simulink model "GCI_Ctrl_PLL_C2000"  (R2024a)
settings: Solver=FixedStepDiscrete  StartTime=0.0  StopTime=8  FixedStep=Sim.ContSampleTime  RelTol=1e-3  EnableMultiTasking=on
values from neighbouring files (symbols this model uses):
  ADPTV = 1.3912    [ModelDD.sldd]
  Ctrl = 0    [ModelDD.sldd]
  EnableMonitors = 0    [ModelDD.sldd]
  FrcPwr = 1    [ModelDD.sldd]
  IdSp = 0.0    [ModelDD.sldd]
  IqSp = 0.0    [ModelDD.sldd]
  ModReq = 1    [ModelDD.sldd]
  PorISel = 0    [ModelDD.sldd]
  PSp = 0.0    [ModelDD.sldd]
  QSp = 0.0    [ModelDD.sldd]
  Sim : value not decoded    [ModelDD.sldd]
  Test = 0    [ModelDD.sldd]
  Var = 650.0    [ModelDD.sldd]
undefined symbols (not defined in the file or in its folder): DiscIntNeverNeededParam, Down, GPTRIP1SEL, GPTRIP2SEL, magnitude, P, TZ1, TZ2, Up
libraries: simulink x38, c2837xDlib x22, c2802xlib x15, slpidlib x9, spsMeanLib x9, spsCurrentMeasurementLib x7, spsThreePhaseVIMeasurementLib x5, spsVoltageMeasurementLib x5, spsTHDLib x4, spsSeriesRLCBranchLib x4, svdutilitieslib x3, c280xlib x3
(part 1 of 11)
settings Model: SimulationMode=accelerator  ExtModeTrigDuration=8  Creator=OmarH  LastModifiedBy=The Professionals
settings SolverCC: AlgebraicLoopSolver=TrustRegion
settings DataIOCC: SaveFormat=StructureWithTime  SaveOutput=off  DSMLogging=off  SaveTime=off
settings OptimizationCC: DefaultParameterBehavior=Inlined  DefaultUnderspecifiedDataType=single  EnhancedBackFolding=on  PassReuseOutputArgsAs=Individual arguments  EfficientMapNaN2IntZero=off  MaxStackSize=1024  OptimizeBlockOrder=speed  DifferentSizesBufferReuse=on  OptimizationCustomize=off  DenormalBehavior=FlushToZero  EfficientTunableParamExpr=on
settings DebuggingCC: MultiTaskDSMMsg=none  ParameterTunabilityLossMsg=error  UnconnectedInputMsg=warning  UnconnectedOutputMsg=warning  UnconnectedLineMsg=warning
settings HardwareCC: ProdBitPerChar=16  ProdBitPerInt=16  ProdBitPerPointer=32  ProdBitPerSizeT=32  ProdBitPerPtrDiffT=32  ProdLargestAtomicInteger=Integer  ProdLargestAtomicFloat=None  ProdWordSize=16  ProdLongLongMode=on  ProdHWDeviceType=Texas Instruments->C2000  TargetBitPerChar=16  TargetBitPerInt=16  TargetLargestAtomicInteger=Integer  TargetIntDivRoundTo=Zero  TargetEndianess=LittleEndian  TargetWordSize=16  TargetHWDeviceType=Texas Instruments->C2000  HardwareBoardFeatureSet=SoCBlockset
settings ModelReferenceCC: EnableRefExpFcnMdlSchedulingChecks=on  ModelReferenceNumInstancesAllowed=Single
settings SFSimCC: MATLABDynamicMemAlloc=off
settings RTWCC: Description=Embedded Coder  SystemTargetFile=ert.tlc  HardwareBoard=TI Delfino F28379D LaunchPad  TemplateMakefile=ert_default_tmf  Toolchain=Texas Instruments Code Composer Studio (C2000)  CodeProfilingSaveOptions=MetricsOnly
settings CodeAppCC: ForceParamTrailComments=on  IgnoreCustomStorageClasses=off  MaxIdLength=128  OperatorAnnotations=on  SimulinkDataObjDesc=on  SFDataObjDesc=on  InsertBlockDesc=on
settings ERTTargetCC: CodeReplacementLibrary=TI C28x  ExtMode=on  ExtModeTransport=4  ExtModeStaticAlloc=on  ExtModeAutomaticAllocSize=off  ExtModeStaticAllocSize=10000  ExtModeMexFile=ext_xcp  ExtModeMexArgs=1 4 5000000  ExtModeIntrfLevel=Level2 - Open

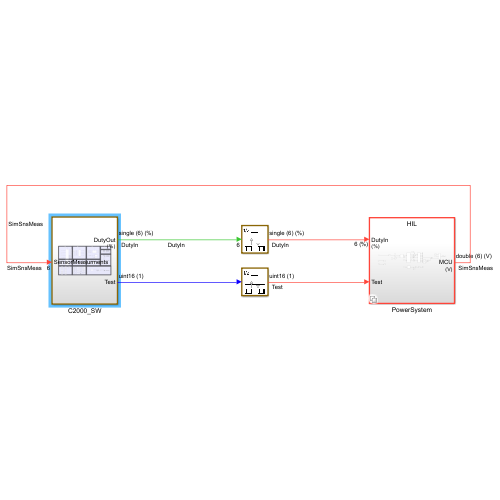
[thumbnail: Simulink's stored preview of the top-level diagram]
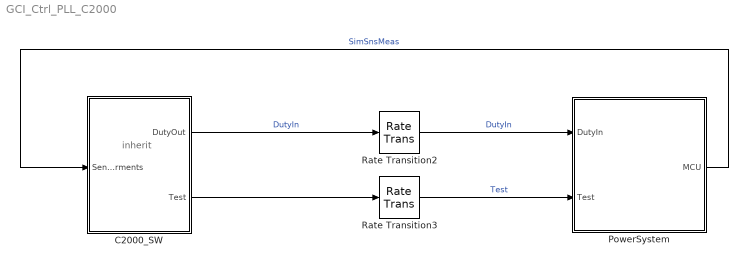
== system GCI_Ctrl_PLL_C2000 ==
  note: inherit
  C2000_SW : Subsystem
  PowerSystem : Subsystem  Variant=on  VariantControl=Variant1
  Rate Transition2 : RateTransition  OutPortSampleTime=Sim.ContSampleTime
  Rate Transition3 : RateTransition  OutPortSampleTime=Sim.ContSampleTime
  wires:
  Rate Transition3/1 -> PowerSystem/2(Test)  "Test"
  C2000_SW/2(Test) -> Rate Transition3/1
  PowerSystem/1(MCU) -> C2000_SW/1(SensorMeasurments)  "SimSnsMeas"
  C2000_SW/1(DutyOut) -> Rate Transition2/1  "DutyIn"
  Rate Transition2/1 -> PowerSystem/1(DutyIn)  "DutyIn"

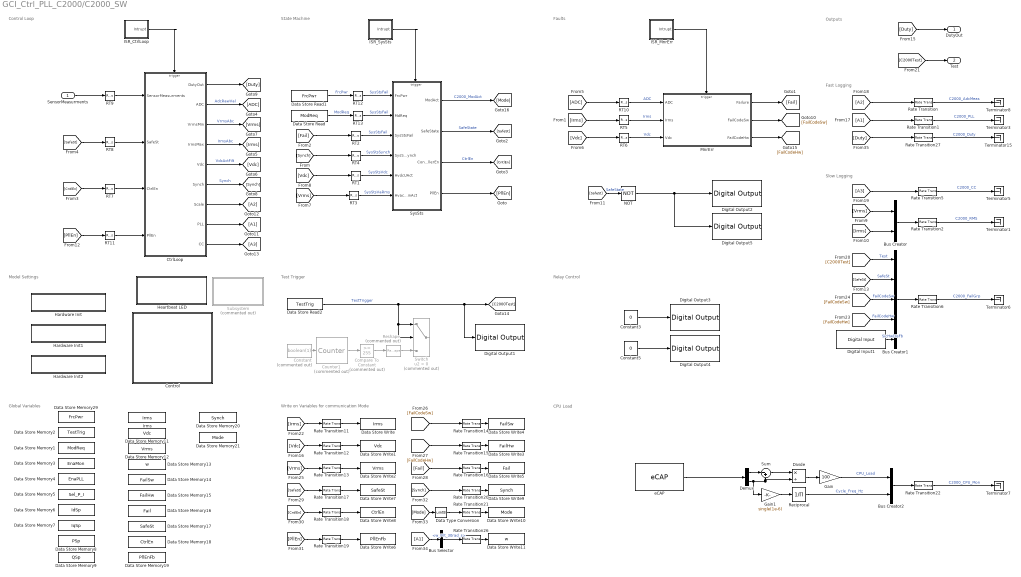
== system GCI_Ctrl_PLL_C2000/C2000_SW ==
  note: Model Settings
  note: Write on Variables for communication Mode
  note: Global Variables
  note: CPU Load
  note: Outputs
  note: Test Trigger
  note: Faults
  note: Relay Control
  note: Control Loop
  note: State Machine
  note: Fast Logging
  note: Slow Logging
  SensorMeasurments : Inport
  Bus Creator : BusCreator  Inputs=2
  Bus Creator1 : BusCreator  Inputs=5
  Bus Creator2 : BusCreator  Inputs=2
  Bus Selector : BusSelector  OutputSignals=w_Filt_30rad_s
  Compare To Constant : simulink/Logic and Bit Operations/Compare To Constant  Commented=on  relop=>=  const=255  OutDataTypeStr=boolean
  Constant : Constant  Commented=on  Value=boolean(1)
  Constant3 : Constant  Value=0  OutDataTypeStr=boolean  SampleTime=10/double(Var.PWM_Freq)
  Constant5 : Constant  Value=0  OutDataTypeStr=boolean  SampleTime=10/double(Var.PWM_Freq)
  Control : Subsystem  Variant=on  VariantControl=Subsystem1
  Counter1 : dspswit3/Counter  Commented=on  Direction=Up  CountEvent=Free running  CounterSize=8 bits  MaxCount=255  InitialCount=0  Output=Count  HitValue=32  ResetInput=on  SamplesPerFrame=1  Ts=1  CntDtype=uint8  HitDtype=Logical
  CtrlLoop : Subsystem
  Data Store Memory1 : DataStoreMemory  DataStoreName=ModReq  WriteAfterWriteMsg=warning  ShowAdditionalParam=off
  Data Store Memory11 : DataStoreMemory  DataStoreName=Vdc  WriteAfterWriteMsg=warning  WriteAfterReadMsg=warning  ShowAdditionalParam=off  OutDataTypeStr=single
  Data Store Memory12 : DataStoreMemory  DataStoreName=Vrms  WriteAfterWriteMsg=warning  WriteAfterReadMsg=warning  ShowAdditionalParam=off  OutDataTypeStr=single
  Data Store Memory13 : DataStoreMemory  DataStoreName=w  WriteAfterWriteMsg=warning  WriteAfterReadMsg=warning  ShowAdditionalParam=off  OutDataTypeStr=single
  Data Store Memory14 : DataStoreMemory  DataStoreName=FailSw  WriteAfterWriteMsg=warning  WriteAfterReadMsg=warning  ShowAdditionalParam=off  OutDataTypeStr=uint16
  Data Store Memory15 : DataStoreMemory  DataStoreName=FailHw  WriteAfterWriteMsg=warning  WriteAfterReadMsg=warning  ShowAdditionalParam=off  OutDataTypeStr=uint8
  Data Store Memory16 : DataStoreMemory  DataStoreName=Fail  WriteAfterWriteMsg=warning  WriteAfterReadMsg=warning  ShowAdditionalParam=off  OutDataTypeStr=boolean
  Data Store Memory17 : DataStoreMemory  DataStoreName=SafeSt  WriteAfterWriteMsg=warning  WriteAfterReadMsg=warning  ShowAdditionalParam=off  OutDataTypeStr=boolean
  Data Store Memory18 : DataStoreMemory  DataStoreName=CtrlEn  WriteAfterWriteMsg=warning  WriteAfterReadMsg=warning  ShowAdditionalParam=off  OutDataTypeStr=boolean
  Data Store Memory19 : DataStoreMemory  DataStoreName=PllEnFb  WriteAfterWriteMsg=warning  WriteAfterReadMsg=warning  ShowAdditionalParam=off  OutDataTypeStr=boolean
  Data Store Memory2 : DataStoreMemory  DataStoreName=TestTrig  WriteAfterWriteMsg=warning  WriteAfterReadMsg=warning  ShowAdditionalParam=off
  Data Store Memory20 : DataStoreMemory  DataStoreName=Synch  WriteAfterWriteMsg=warning  WriteAfterReadMsg=warning  ShowAdditionalParam=off  OutDataTypeStr=boolean
  Data Store Memory21 : DataStoreMemory  DataStoreName=Mode  WriteAfterWriteMsg=warning  WriteAfterReadMsg=warning  ShowAdditionalParam=off  OutDataTypeStr=uint8
  Data Store Memory29 : DataStoreMemory  DataStoreName=FrcPwr  WriteAfterWriteMsg=warning  ShowAdditionalParam=off
  Data Store Memory3 : DataStoreMemory  DataStoreName=EnaMon  ShowAdditionalParam=off
  Data Store Memory4 : DataStoreMemory  DataStoreName=EnaPLL  WriteAfterWriteMsg=warning  WriteAfterReadMsg=warning  ShowAdditionalParam=off  OutDataTypeStr=boolean
  Data Store Memory5 : DataStoreMemory  DataStoreName=Sel_P_I  ShowAdditionalParam=off
  Data Store Memory6 : DataStoreMemory  DataStoreName=IdSp  ShowAdditionalParam=off  OutDataTypeStr=single
  Data Store Memory7 : DataStoreMemory  DataStoreName=IqSp  ShowAdditionalParam=off  OutDataTypeStr=single
  Data Store Memory8 : DataStoreMemory  DataStoreName=PSp  WriteAfterWriteMsg=warning  ShowAdditionalParam=off  OutDataTypeStr=single
  Data Store Memory9 : DataStoreMemory  DataStoreName=QSp  WriteAfterWriteMsg=warning  ShowAdditionalParam=off  OutDataTypeStr=single
  Data Store Read : DataStoreRead  DataStoreName=ModReq  SampleTime=10/double(Var.PWM_Freq)  IndexOptions=Index vector (dialog)  Indices=1  OutputSizes=1
  Data Store Read1 : DataStoreRead  DataStoreName=FrcPwr  SampleTime=10/double(Var.PWM_Freq)  IndexOptions=Index vector (dialog)  Indices=1  OutputSizes=1
  Data Store Read2 : DataStoreRead  DataStoreName=TestTrig  SampleTime=10/double(Var.PWM_Freq)  IndexOptions=Index vector (dialog)  Indices=1  OutputSizes=1
  Data Store Write : DataStoreWrite  DataStoreName=Irms  IndexOptions=Index vector (dialog)  Indices=1  OutputSizes=1
  Data Store Write1 : DataStoreWrite  DataStoreName=Vdc  IndexOptions=Index vector (dialog)  Indices=1  OutputSizes=1
  Data Store Write10 : DataStoreWrite  DataStoreName=Mode  IndexOptions=Index vector (dialog)  Indices=1  OutputSizes=1
  Data Store Write11 : DataStoreWrite  DataStoreName=w  IndexOptions=Index vector (dialog)  Indices=1  OutputSizes=1
  Data Store Write2 : DataStoreWrite  DataStoreName=Vrms  IndexOptions=Index vector (dialog)  Indices=1  OutputSizes=1
  Data Store Write3 : DataStoreWrite  DataStoreName=FailHw  IndexOptions=Index vector (dialog)  Indices=1  OutputSizes=1
  Data Store Write4 : DataStoreWrite  DataStoreName=FailSw  IndexOptions=Index vector (dialog)  Indices=1  OutputSizes=1
  Data Store Write5 : DataStoreWrite  DataStoreName=Fail  IndexOptions=Index vector (dialog)  Indices=1  OutputSizes=1
  Data Store Write6 : DataStoreWrite  DataStoreName=PllEnFb  IndexOptions=Index vector (dialog)  Indices=1  OutputSizes=1
  Data Store Write7 : DataStoreWrite  DataStoreName=SafeSt  IndexOptions=Index vector (dialog)  Indices=1  OutputSizes=1
  Data Store Write8 : DataStoreWrite  DataStoreName=CtrlEn  IndexOptions=Index vector (dialog)  Indices=1  OutputSizes=1
  Data Store Write9 : DataStoreWrite  DataStoreName=Synch  IndexOptions=Index vector (dialog)  Indices=1  OutputSizes=1
  Data Type Conversion : DataTypeConversion  OutDataTypeStr=uint8  SaturateOnIntegerOverflow=off  RndMeth=Floor
  Demux : Demux  Outputs=2
  Digital Input1 : c2837xDlib/Digital Input  GPIO_Number=GPIO88~GPIO95  GPIO_Bit0=off  GPIO_Bit1=off  GPIO_Bit2=off  GPIO_Bit3=off  GPIO_Bit4=off  GPIO_Bit5=off  GPIO_Bit6=on  GPIO_Bit7=off  sampleTime=10/double(Var.PWM_Freq)  dataType=boolean  GPIO_Bit0_Qualification=Sync to SYSCLKOUT  GPIO_Bit1_Qualification=Sync to SYSCLKOUT  GPIO_Bit2_Qualification=Sync to SYSCLKOUT  GPIO_Bit3_Qualification=Sync to SYSCLKOUT  GPIO_Bit4_Qualification=Sync to SYSCLKOUT  GPIO_Bit5_Qualification=Sync to SYSCLKOUT  GPIO_Bit6_Qualification=Sync to SYSCLKOUT  GPIO_Bit7_Qualification=Sync to SYSCLKOUT  Qualification_Period=-1
  Digital Output1 : c2837xDlib/Digital Output  GPIO_Number=GPIO64~GPIO71  GPIO_Bit0=off  GPIO_BIT0_Toggle=off  GPIO_Bit1=off  GPIO_BIT1_Toggle=off  GPIO_Bit2=off  GPIO_BIT2_Toggle=off  GPIO_Bit3=on  GPIO_BIT3_Toggle=off  GPIO_Bit4=off  GPIO_BIT4_Toggle=off  GPIO_Bit5=off  GPIO_BIT5_Toggle=off  GPIO_Bit6=off  GPIO_BIT6_Toggle=off  GPIO_Bit7=off  GPIO_BIT7_Toggle=off
  Digital Output2 : c2837xDlib/Digital Output  GPIO_Number=GPIO8~GPIO15  GPIO_Bit0=off  GPIO_BIT0_Toggle=off  GPIO_Bit1=off  GPIO_BIT1_Toggle=off  GPIO_Bit2=off  GPIO_BIT2_Toggle=off  GPIO_Bit3=off  GPIO_BIT3_Toggle=off  GPIO_Bit4=on  GPIO_BIT4_Toggle=off  GPIO_Bit5=off  GPIO_BIT5_Toggle=off  GPIO_Bit6=off  GPIO_BIT6_Toggle=off  GPIO_Bit7=off  GPIO_BIT7_Toggle=off
  Digital Output3 : c2837xDlib/Digital Output  GPIO_Number=GPIO16~GPIO23  GPIO_Bit0=off  GPIO_BIT0_Toggle=off  GPIO_Bit1=off  GPIO_BIT1_Toggle=off  GPIO_Bit2=on  GPIO_BIT2_Toggle=off  GPIO_Bit3=off  GPIO_BIT3_Toggle=off  GPIO_Bit4=off  GPIO_BIT4_Toggle=off  GPIO_Bit5=off  GPIO_BIT5_Toggle=off  GPIO_Bit6=off  GPIO_BIT6_Toggle=off  GPIO_Bit7=off  GPIO_BIT7_Toggle=off
  Digital Output4 : c2837xDlib/Digital Output  GPIO_Number=GPIO16~GPIO23  GPIO_Bit0=off  GPIO_BIT0_Toggle=off  GPIO_Bit1=off  GPIO_BIT1_Toggle=off  GPIO_Bit2=off  GPIO_BIT2_Toggle=off  GPIO_Bit3=on  GPIO_BIT3_Toggle=off  GPIO_Bit4=off  GPIO_BIT4_Toggle=off  GPIO_Bit5=off  GPIO_BIT5_Toggle=off  GPIO_Bit6=off  GPIO_BIT6_Toggle=off  GPIO_Bit7=off  GPIO_BIT7_Toggle=off
  Digital Output5 : c2837xDlib/Digital Output  GPIO_Number=GPIO8~GPIO15  GPIO_Bit0=off  GPIO_BIT0_Toggle=off  GPIO_Bit1=off  GPIO_BIT1_Toggle=off  GPIO_Bit2=off  GPIO_BIT2_Toggle=off  GPIO_Bit3=off  GPIO_BIT3_Toggle=off  GPIO_Bit4=off  GPIO_BIT4_Toggle=off  GPIO_Bit5=off  GPIO_BIT5_Toggle=off  GPIO_Bit6=on  GPIO_BIT6_Toggle=off  GPIO_Bit7=off  GPIO_BIT7_Toggle=off
  Divide : Product  Inputs=*/
  Gain : Gain  Gain=100
  Gain1 : Gain  Gain=single(1e-6)  ParamDataTypeStr=single
  Hardware Init : Subsystem  TreatAsAtomicUnit=on
  Hardware Init1 : Subsystem  TreatAsAtomicUnit=on
  Hardware Init2 : Subsystem  TreatAsAtomicUnit=on
  Heartbeat LED : Subsystem
  ISR_CtrlLoop : Subsystem  Variant=on  VariantControl=Variant1
  ISR_MnrErr : Subsystem  Variant=on  VariantControl=Variant1
  ISR_SysSts : Subsystem  Variant=on  VariantControl=Variant1
  Irms : DataStoreMemory  DataStoreName=Irms  WriteAfterWriteMsg=warning  WriteAfterReadMsg=warning  ShowAdditionalParam=off  OutDataTypeStr=single
  MnrErr : Subsystem
  NOT : Logic  Operator=NOT  IconShape=distinctive  AllPortsSameDT=off  OutDataTypeStr=boolean
  RT{1..13} (13 alike) : RateTransition  Deterministic=off  OutPortSampleTimeOpt=Inherit  OutPortSampleTime=0.001
  Rate Transition : RateTransition  Deterministic=off  OutPortSampleTime=Sim.MeasFastSmplTime
  Rate Transition1 : RateTransition  Deterministic=off  OutPortSampleTime=Sim.MeasFastSmplTime
  Rate Transition{2,5..6,11..22,26} (16 alike) : RateTransition  Deterministic=off  OutPortSampleTime=Sim.MeasSlowSmplTime
  Rate Transition27 : RateTransition  Deterministic=off  OutPortSampleTime=Sim.MeasFastSmplTime
  Reciprocal : Product  Inputs=/
  Reshape : Reshape  Commented=on
  Subsystem : Subsystem  Commented=on
  Sum : Sum  Inputs=|-+
  Switch : Switch  Commented=on  Criteria=u2 > Threshold  SaturateOnIntegerOverflow=off  InputSameDT=off
  SysSts : Subsystem
  Terminator{1,3,5..8,15} (7 alike) : Terminator
  eCAP : c280xlib/eCAP  operatingMode=eCAP  selectCAPx=eCAP1  offsetValue=0  counterSynIn=off  enableCounter=off  syncOutput=Disabled  sampleTime=1/1000  eventPrescaler=0  HREnable=off  continuousCalibration=off  calibrationPeriod=0.0016  selectMode=Continuous  enableOneShot=off  stopValue=Capture Event 2  resetEv1Ts=off  ev1Polarity=Rising Edge  resetEv2Ts=on  ev2Polarity=Falling Edge  resetEv3Ts=off  ev3Polarity=Rising Edge  resetEv4Ts=off  ev4Polarity=Rising Edge  outputType=Microseconds  tSCntrDataType=single  capEvFlag=off  capFlagDataType=uint16  overFlowFlag=off  overFlowFlagDataType=uint16  periodUnit=Seconds  periodSource=Specify via dialog  waveformPeriod=0.001  dutyUnit=Percentages  dutySource=Specify via dialog  dutyCycle=50  outputPolarity=Active High  enableCEVT1Int=off  enableCEVT2Int=off  enableCEVT3Int=off  enableCEVT4Int=off  enableCTROVFInt=off  enablePRDInt=off  enableCMPInt=off
      settings: LibrarySourceBlock=c2837xDlib/eCAP
  DutyOut : Outport  Unit=%
  Test : Outport  Port=2
  wires:
  ISR_CtrlLoop/1(Intrupt) -> CtrlLoop/Trigger
  ISR_SysSts/1(Intrupt) -> SysSts/Trigger
  MnrErr/1(Failure) -> [Fail]
  Data Store Read/1 -> RT13/1  "ModReq"
  [SafeSt] -> RT8/1
  [CntlEn] -> RT7/1
  ISR_MnrErr/1(Intrupt) -> MnrErr/Trigger
  CtrlLoop/2(ADC) -> [ADC]  "AdcRawVal"
  CtrlLoop/4(IrmsMax) -> [Irms]  "IrmsAbc"
  [Irms] -> RT5/1
  [Vdc] -> RT6/1
  CtrlLoop/3(VrmsMin) -> [Vrms]  "VrmsAbc"
  RT3/1 -> SysSts/6(HvacUMinAct)  "SysStsVaRms"
  [Vrms] -> RT3/1
  [Vdc] -> RT1/1
  [Fail] -> RT2/1
  RT10/1 -> MnrErr/1(ADC)  "ADC"
  RT5/1 -> MnrErr/2(Irms)  "Irms"
  RT6/1 -> MnrErr/3(Vdc)  "Vdc"
  CtrlLoop/6(Synch) -> [Synch]  "Synch"
  [Synch] -> RT4/1
  Data Store Read1/1 -> RT12/1  "FrcPwr"
  [ADC] -> RT10/1
  RT4/1 -> SysSts/4(SysStsSynch)  "SysStsSynch"
  RT1/1 -> SysSts/5(HvdcUAct)  "SysStsVdc"
  RT2/1 -> SysSts/3(SysStsFail)  "SysStsFail"
  SysSts/2(SafeState) -> [SafeSt]  "SafeState"
  SysSts/3(ControllerEn) -> [CntlEn]  "CtrlEn"
  CtrlLoop/5(Vdc) -> [Vdc]  "VdcActFilt"
  Rate Transition/1 -> Terminator8/1  "C2000_AdcMeas"
  Rate Transition1/1 -> Terminator3/1  "C2000_PLL"
  Rate Transition2/1 -> Terminator1/1  "C2000_RMS"
  CtrlLoop/1(DutyOut) -> [Duty]
  Rate Transition5/1 -> Terminator5/1  "C2000_CC"
  Counter1/1 -> Compare To Constant/1
  Compare To Constant/1 -> Reshape/1
  Rate Transition6/1 -> Terminator6/1  "C2000_FailGrp"
  RT7/1 -> CtrlLoop/3(CtrlEn)
  RT8/1 -> CtrlLoop/2(SafeSt)
  [SafeSt] -> NOT/1  "SafeState"
  SensorMeasurments/1 -> RT9/1
  RT9/1 -> CtrlLoop/1(SensorMeasurments)
  SysSts/1(ModAct) -> [Mode]  "C2000_ModAct"
  RT11/1 -> CtrlLoop/4(PllEn)
  [PllEn] -> RT11/1
  SysSts/4(PllEn) -> [PllEn]
  Reshape/1 -> Switch/3
  [Duty] -> DutyOut/1
  CtrlLoop/8(PLL) -> [A1]
  [A1] -> Rate Transition1/1
  CtrlLoop/7(" Scale") -> [A2]
  [A2] -> Rate Transition/1
  CtrlLoop/9(CC) -> [A3]
  [A3] -> Rate Transition5/1
  [C2000Test] -> Test/1
  MnrErr/2(FailCodeSw) -> [FailCodeSw]
  Constant5/1 -> Digital Output4/1
  Constant3/1 -> Digital Output3/1
  MnrErr/3(FailCodeHw) -> [FailCodeHw]
  NOT/1 -> Digital Output5/1, Digital Output2/1
  Constant/1 -> Counter1/1
  Rate Transition22/1 -> Terminator7/1  "C2000_CPU_Mon"
  eCAP/1 -> Demux/1
  Demux/1 -> Sum/1
  Demux/2 -> Gain1/1, Sum/2, Divide/2
  Sum/1 -> Divide/1
  Divide/1 -> Gain/1
  Gain/1 -> Bus Creator2/1  "CPU_Load"
  Reciprocal/1 -> Bus Creator2/2  "Cycle_Freq_Hz"
  Gain1/1 -> Reciprocal/1
  Data Store Read2/1 -> Switch/1, Switch/2, Digital Output1/1, [C2000Test]  "TestTrigger"
  Rate Transition21/1 -> Data Store Write10/1
  [CntlEn] -> Rate Transition18/1
  [FailCodeHw] -> Rate Transition15/1
  [Synch] -> Rate Transition20/1
  [PllEn] -> Rate Transition19/1
  Rate Transition18/1 -> Data Store Write8/1
  Rate Transition19/1 -> Data Store Write6/1
  [FailCodeSw] -> Rate Transition14/1
  Rate Transition16/1 -> Data Store Write5/1
  [SafeSt] -> Rate Transition17/1
  Rate Transition14/1 -> Data Store Write4/1
  [Mode] -> Data Type Conversion/1
  Rate Transition20/1 -> Data Store Write9/1
  Rate Transition17/1 -> Data Store Write7/1
  Rate Transition15/1 -> Data Store Write3/1
  Rate Transition12/1 -> Data Store Write1/1
  Rate Transition11/1 -> Data Store Write/1
  [Vrms] -> Rate Transition13/1
  Data Type Conversion/1 -> Rate Transition21/1
  Rate Transition13/1 -> Data Store Write2/1
  [Fail] -> Rate Transition16/1
  [Vdc] -> Rate Transition12/1
  [Irms] -> Rate Transition11/1
  Bus Selector/1 -> Rate Transition26/1  "<w_Filt_30rad_s>"
  [A1] -> Bus Selector/1
  Rate Transition26/1 -> Data Store Write11/1
  Rate Transition27/1 -> Terminator15/1  "C2000_Duty"
  [Duty] -> Rate Transition27/1
  [Irms] -> Bus Creator/2
  [Vrms] -> Bus Creator/1
  Bus Creator/1 -> Rate Transition2/1
  Digital Input1/1 -> Bus Creator1/5  "SicHwDisFb"
  [FailCodeHw] -> Bus Creator1/4  "FailCodeHw"
  [FailCodeSw] -> Bus Creator1/3  "FailCodeSw"
  [SafeSt] -> Bus Creator1/2  "SafeSt"
  [C2000Test] -> Bus Creator1/1  "Test"
  Bus Creator1/1 -> Rate Transition6/1
  Bus Creator2/1 -> Rate Transition22/1
  RT12/1 -> SysSts/1(FrcPwr)  "SysStsFail"
  RT13/1 -> SysSts/2(MdReq)  "SysStsFail"

== system GCI_Ctrl_PLL_C2000/PowerSystem ==
  DutyIn : Inport  Unit=%
  Test : Inport  Port=2
  Actual System : Subsystem  VariantControl="Sim.PlantOrMeas == \"ActPlant\""
  HIL : Subsystem  VariantControl="Sim.PlantOrMeas == \"HIL\""  ReferencedSubsystem=HIL
  HW : Subsystem  VariantControl="Sim.PlantOrMeas ==\"HW\""
  Meas : Subsystem  VariantControl="Sim.PlantOrMeas == \"Measurments\""
  Plant : Subsystem  VariantControl="Sim.PlantOrMeas == \"Plant\""
  MCU : Outport  Unit=V  VectorParamsAs1DForOutWhenUnconnected=off

== system GCI_Ctrl_PLL_C2000/C2000_SW/Control ==
  CommunicationMode : Subsystem  VariantControl="Sim.ExternalOrComm == \"Comm\""
  ExternalMode : Subsystem  VariantControl="Sim.ExternalOrComm == \"External\""

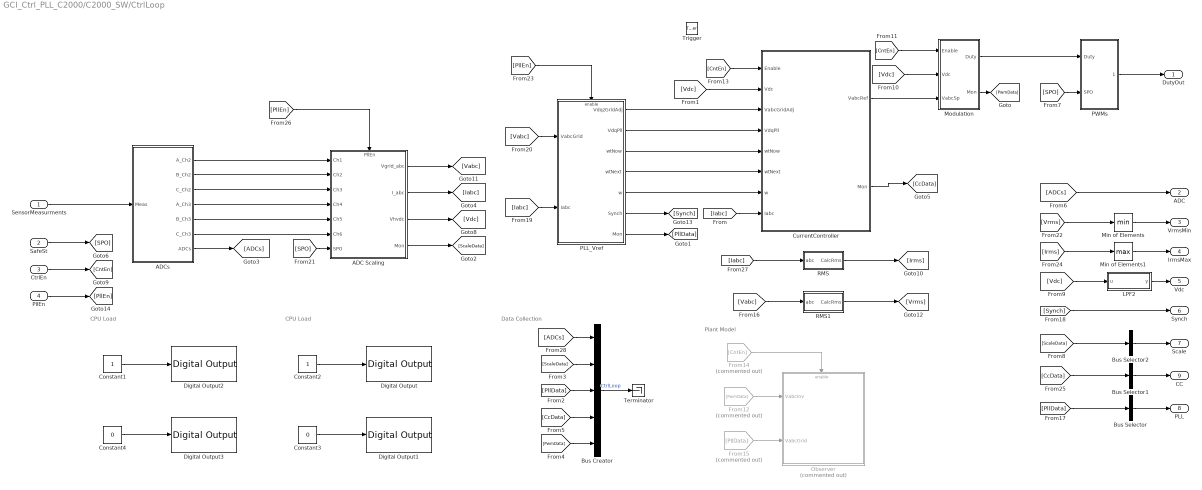
== system GCI_Ctrl_PLL_C2000/C2000_SW/CtrlLoop ==
  note: Plant Model
  note: Data Collection
  note: CPU Load
  note: CPU Load
  SensorMeasurments : Inport
  SafeSt : Inport  Port=2
  CtrlEn : Inport  Port=3
  PllEn : Inport  Port=4
  Trigger : TriggerPort  TriggerType=function-call  VariantControl=Variant  PortDimensions=1  OutDataTypeStr=single
  ADC Scaling : Subsystem  Priority=2  Variant=on  VariantControl=Variant1
      settings: PortSchema="{\"entries\":[{\"content\":{\"sides\":[{\"content\":{\"connectorIds\":[\"In1\",\"In2\",\"In3\",\"In4\",\"In5\",\"In6\",\"In7\"]},\"type\":\"ConnectorPlacement.EquallySpacedRectSide\",\"uuid\":\"8934cdca-9946-4b97-8ba4-78519e8d05cc\"},{\"content\":{\"connectorIds\":[\"Out1\",\"Out2\",\"Out3\",\"Out4\"],\"side\":\"RIGHT\"},\"type\":\"ConnectorPlacement.EquallySpacedRectSide\",\"uuid\":\"2243c45a-8cb3-4bd7-a41f-11141637ae25\"},{\"content\":{\"connectorIds\":[\"In8\"],\"side\":\"TOP\"},\"type\":\"ConnectorPlacement.EquallySpacedRectSide\",\"uuid\":\"be0bda9a-60e5-46f8-8e85-9e009f5b84ca\"}]},\"type\":\"ConnectorPlacement.EquallySpacedConnector\",\"uuid\":\"8d50c192-10ab-4db2-830e-ba02c49e8fdf\"}],\"packageUris\":[\"http://schema.mathworks.com/mf0/Connector/R2020b\"],\"version\":\"1.0\"}"
  ADCs : Subsystem  Priority=2  Variant=on  VariantControl=Variant1
  Bus Creator : BusCreator  Inputs=5
  Bus Selector : BusSelector  OutputSignals=Vdqz,Vdqz_Pll,Idqz,PQ,wtCur,w,w_Filt_30rad_s,VgQSynch,VabcGridAdj,wtNext  OutputAsBus=on
  Bus Selector1 : BusSelector  OutputSignals=IdqzRef,VdqPRef,PQRef  OutputAsBus=on
  Bus Selector2 : BusSelector  OutputSignals=VaActMeas,VbActMeas,IaActMeas,IbActMeas,IcActMeas,VdcActMeas,Vabc_NoDcOff,Iabc_NoDcOff  OutputAsBus=on
  Constant1 : Constant  Priority=1  OutDataTypeStr=boolean
  Constant2 : Constant  Priority=1  OutDataTypeStr=boolean
  Constant3 : Constant  Priority=3  Value=0  OutDataTypeStr=boolean
  Constant4 : Constant  Priority=3  Value=0  OutDataTypeStr=boolean
  CurrentController : Subsystem  Priority=2  Variant=on  VariantControl=Variant1
  Digital Output : c2837xDlib/Digital Output  Priority=1  GPIO_Number=GPIO64~GPIO71  GPIO_Bit0=off  GPIO_BIT0_Toggle=off  GPIO_Bit1=off  GPIO_BIT1_Toggle=off  GPIO_Bit2=on  GPIO_BIT2_Toggle=off  GPIO_Bit3=off  GPIO_BIT3_Toggle=off  GPIO_Bit4=off  GPIO_BIT4_Toggle=off  GPIO_Bit5=off  GPIO_BIT5_Toggle=off  GPIO_Bit6=off  GPIO_BIT6_Toggle=off  GPIO_Bit7=off  GPIO_BIT7_Toggle=off
  Digital Output1 : c2837xDlib/Digital Output  Priority=3  GPIO_Number=GPIO64~GPIO71  GPIO_Bit0=off  GPIO_BIT0_Toggle=off  GPIO_Bit1=off  GPIO_BIT1_Toggle=off  GPIO_Bit2=on  GPIO_BIT2_Toggle=off  GPIO_Bit3=off  GPIO_BIT3_Toggle=off  GPIO_Bit4=off  GPIO_BIT4_Toggle=off  GPIO_Bit5=off  GPIO_BIT5_Toggle=off  GPIO_Bit6=off  GPIO_BIT6_Toggle=off  GPIO_Bit7=off  GPIO_BIT7_Toggle=off
  Digital Output2 : c2837xDlib/Digital Output  Priority=1  GPIO_Number=GPIO16~GPIO23  GPIO_Bit0=off  GPIO_BIT0_Toggle=off  GPIO_Bit1=off  GPIO_BIT1_Toggle=off  GPIO_Bit2=off  GPIO_BIT2_Toggle=off  GPIO_Bit3=off  GPIO_BIT3_Toggle=off  GPIO_Bit4=on  GPIO_BIT4_Toggle=off  GPIO_Bit5=off  GPIO_BIT5_Toggle=off  GPIO_Bit6=off  GPIO_BIT6_Toggle=off  GPIO_Bit7=off  GPIO_BIT7_Toggle=off
  Digital Output3 : c2837xDlib/Digital Output  Priority=3  GPIO_Number=GPIO16~GPIO23  GPIO_Bit0=off  GPIO_BIT0_Toggle=off  GPIO_Bit1=off  GPIO_BIT1_Toggle=off  GPIO_Bit2=off  GPIO_BIT2_Toggle=off  GPIO_Bit3=off  GPIO_BIT3_Toggle=off  GPIO_Bit4=on  GPIO_BIT4_Toggle=off  GPIO_Bit5=off  GPIO_BIT5_Toggle=off  GPIO_Bit6=off  GPIO_BIT6_Toggle=off  GPIO_Bit7=off  GPIO_BIT7_Toggle=off
  From12 : From  Commented=on  GotoTag=PwmData
  From14 : From  Commented=on  GotoTag=CntEn
  From15 : From  Commented=on  GotoTag=PllData
  LPF2 : Subsystem  Priority=2  mask{Ts=1/(Var.PWM_Freq), w=single(2*pi*10), K=single(1), y_0=single(0)}
      mask prompts: Ts "Sample Time (s)"; w "CutOff Freq (-3db) (rad/s)"; K "Gain"; y_0 "Initial output"
  Min of Elements : MinMax  Priority=2
  Min of Elements1 : MinMax  Priority=2  Function=max
  Modulation : Subsystem  Priority=2  Variant=on  VariantControl=Variant1
  Observer : Subsystem  Priority=2  Commented=on
  PLL_Vref : Subsystem  Priority=2
  PWMs : Subsystem  Priority=2  Variant=on  VariantControl=Variant1
  RMS : Subsystem  Priority=2
  RMS1 : Subsystem  Priority=2
  Terminator : Terminator
  DutyOut : Outport  OutDataTypeStr=single  VectorParamsAs1DForOutWhenUnconnected=off
  ADC : Outport  Port=2  VectorParamsAs1DForOutWhenUnconnected=off
  VrmsMin : Outport  Port=3  Unit=V  VectorParamsAs1DForOutWhenUnconnected=off
  IrmsMax : Outport  Port=4  Unit=A  VectorParamsAs1DForOutWhenUnconnected=off
  Vdc : Outport  Port=5  Unit=V  VectorParamsAs1DForOutWhenUnconnected=off
  Synch : Outport  Port=6  VectorParamsAs1DForOutWhenUnconnected=off
  " Scale" : Outport  Port=7
  PLL : Outport  Port=8
  CC : Outport  Port=9
  wires:
  Constant3/1 -> Digital Output1/1
  Constant2/1 -> Digital Output/1
  PLL_Vref/4(wtNext) -> CurrentController/6(wtNext)
  Modulation/1(Duty) -> PWMs/1(Duty)
  SensorMeasurments/1 -> ADCs/1(Meas)
  Modulation/2(Mon) -> [PwmData]
  PLL_Vref/5(w) -> CurrentController/7(w)
  CurrentController/2(Mon) -> [CcData]
  [SPO] -> PWMs/2(SPO)
  PWMs/1(DutyOut) -> DutyOut/1
  CurrentController/1(VabcRef) -> Modulation/3(VabcSp)
  ADC Scaling/1(Vgrid_abc) -> [Vabc]
  ADC Scaling/2(I_abc) -> [Iabc]
  ADCs/1(A_Ch2) -> ADC Scaling/1(Ch1)
  ADCs/2(B_Ch2) -> ADC Scaling/2(Ch2)
  ADCs/3(C_Ch2) -> ADC Scaling/3(Ch3)
  ADCs/4(A_Ch3) -> ADC Scaling/4(Ch4)
  ADCs/5(B_Ch3) -> ADC Scaling/5(Ch5)
  PLL_Vref/1(VdqzGridAdj) -> CurrentController/3(VabcGridAdj)
  ADCs/6(C_Ch3) -> ADC Scaling/6(Ch6)
  ADC Scaling/3(Vhvdc) -> [Vdc]
  [Vdc] -> Modulation/2(Vdc)
  [CntEn] -> CurrentController/1(Enable)
  [CntEn] -> Modulation/1(Enable)
  From12/1 -> Observer/1(VabcInv)
  From15/1 -> Observer/2(VabcGrid)
  From14/1 -> Observer/Enable
  SafeSt/1 -> [SPO]
  CtrlEn/1 -> [CntEn]
  [ADCs] -> ADC/1
  [Iabc] -> CurrentController/8(Iabc)
  RMS/1(CalcRms) -> [Irms]
  Min of Elements1/1 -> IrmsMax/1
  [Vdc] -> LPF2/1(u)
  RMS1/1(CalcRms) -> [Vrms]
  [Vabc] -> RMS1/1(abc)
  Min of Elements/1 -> VrmsMin/1
  PLL_Vref/6(Synch) -> [Synch]
  [Synch] -> Synch/1
  LPF2/1(y) -> Vdc/1
  PLL_Vref/3(wtNow) -> CurrentController/5(wtNow)
  [PllEn] -> PLL_Vref/Enable
  ADC Scaling/4(Mon) -> [ScaleData]
  PLL_Vref/7(Mon) -> [PllData]
  Bus Selector/1 -> PLL/1
  Bus Selector1/1 -> CC/1
  [Iabc] -> PLL_Vref/2(Iabc)
  [Vabc] -> PLL_Vref/1(VabcGrid)
  [SPO] -> ADC Scaling/7(SPO)
  PllEn/1 -> [PllEn]
  [Vrms] -> Min of Elements/1
  [Irms] -> Min of Elements1/1
  [ScaleData] -> Bus Selector2/1
  [PllData] -> Bus Selector/1
  [CcData] -> Bus Selector1/1
  [PllEn] -> ADC Scaling/8(PllEn)
  [Iabc] -> RMS/1(abc)
  PLL_Vref/2(VdqPll) -> CurrentController/4(VdqPll)
  Constant1/1 -> Digital Output2/1
  Constant4/1 -> Digital Output3/1
  ADCs/7(ADCs) -> [ADCs]
  [PwmData] -> Bus Creator/5
  [CcData] -> Bus Creator/4
  [PllData] -> Bus Creator/3
  [ScaleData] -> Bus Creator/2
  [ADCs] -> Bus Creator/1
  Bus Creator/1 -> Terminator/1  "CtrlLoop"
  Bus Selector2/1 -> " Scale"/1
  [Vdc] -> CurrentController/2(Vdc)

== system GCI_Ctrl_PLL_C2000/C2000_SW/Hardware Init ==
  Constant : Constant  Value=0
  Digital Output2 : c2837xDlib/Digital Output  GPIO_Number=GPIO8~GPIO15  GPIO_Bit0=off  GPIO_BIT0_Toggle=off  GPIO_Bit1=off  GPIO_BIT1_Toggle=off  GPIO_Bit2=off  GPIO_BIT2_Toggle=off  GPIO_Bit3=off  GPIO_BIT3_Toggle=off  GPIO_Bit4=on  GPIO_BIT4_Toggle=off  GPIO_Bit5=off  GPIO_BIT5_Toggle=off  GPIO_Bit6=off  GPIO_BIT6_Toggle=off  GPIO_Bit7=off  GPIO_BIT7_Toggle=off
  Event Listener : EventListener  DisableCoverage=on  EventName=reset
  wires:
  Constant/1 -> Digital Output2/1

== system GCI_Ctrl_PLL_C2000/C2000_SW/Hardware Init1 ==
  Constant : Constant  Value=0
  Digital Output2 : c2837xDlib/Digital Output  GPIO_Number=GPIO8~GPIO15  GPIO_Bit0=off  GPIO_BIT0_Toggle=off  GPIO_Bit1=off  GPIO_BIT1_Toggle=off  GPIO_Bit2=off  GPIO_BIT2_Toggle=off  GPIO_Bit3=off  GPIO_BIT3_Toggle=off  GPIO_Bit4=on  GPIO_BIT4_Toggle=off  GPIO_Bit5=off  GPIO_BIT5_Toggle=off  GPIO_Bit6=off  GPIO_BIT6_Toggle=off  GPIO_Bit7=off  GPIO_BIT7_Toggle=off
  Event Listener : EventListener  DisableCoverage=on  EventType=Reset  EventName=reset
  wires:
  Constant/1 -> Digital Output2/1

== system GCI_Ctrl_PLL_C2000/C2000_SW/Hardware Init2 ==
  Constant : Constant  Value=0
  Digital Output2 : c2837xDlib/Digital Output  GPIO_Number=GPIO8~GPIO15  GPIO_Bit0=off  GPIO_BIT0_Toggle=off  GPIO_Bit1=off  GPIO_BIT1_Toggle=off  GPIO_Bit2=off  GPIO_BIT2_Toggle=off  GPIO_Bit3=off  GPIO_BIT3_Toggle=off  GPIO_Bit4=on  GPIO_BIT4_Toggle=off  GPIO_Bit5=off  GPIO_BIT5_Toggle=off  GPIO_Bit6=off  GPIO_BIT6_Toggle=off  GPIO_Bit7=off  GPIO_BIT7_Toggle=off
  Event Listener : EventListener  DisableCoverage=on  EventType=Terminate  EventName=reset
  wires:
  Constant/1 -> Digital Output2/1

== system GCI_Ctrl_PLL_C2000/C2000_SW/Heartbeat LED ==
  note: Heart Rate 1Hz
  Constant : Constant  OutDataTypeStr=boolean  SampleTime=0.5
  Digital Output : c2837xDlib/Digital Output  GPIO_Number=GPIO24~GPIO31  GPIO_Bit0=off  GPIO_BIT0_Toggle=off  GPIO_Bit1=off  GPIO_BIT1_Toggle=off  GPIO_Bit2=off  GPIO_BIT2_Toggle=off  GPIO_Bit3=off  GPIO_BIT3_Toggle=off  GPIO_Bit4=off  GPIO_BIT4_Toggle=off  GPIO_Bit5=off  GPIO_BIT5_Toggle=off  GPIO_Bit6=off  GPIO_BIT6_Toggle=off  GPIO_Bit7=on  GPIO_BIT7_Toggle=on
  wires:
  Constant/1 -> Digital Output/1  "HeartRateEn"

== system GCI_Ctrl_PLL_C2000/C2000_SW/ISR_CtrlLoop ==
  HW : Subsystem  VariantControl="Sim.SimOrHw ==  \"Hw\""
  SIM : Subsystem  VariantControl="Sim.SimOrHw == \"Sim\""
  Intrupt : Outport  VectorParamsAs1DForOutWhenUnconnected=off  OutputFunctionCall=on

== system GCI_Ctrl_PLL_C2000/C2000_SW/ISR_MnrErr ==
  HW : Subsystem  VariantControl="Sim.SimOrHw ==  \"Hw\""
  SIM : Subsystem  VariantControl="Sim.SimOrHw == \"Sim\""
  Intrupt : Outport  VectorParamsAs1DForOutWhenUnconnected=off  OutputFunctionCall=on

== system GCI_Ctrl_PLL_C2000/C2000_SW/ISR_SysSts ==
  HW : Subsystem  VariantControl="Sim.SimOrHw ==  \"Hw\""
  SIM : Subsystem  VariantControl="Sim.SimOrHw == \"Sim\""
  Intrupt : Outport  VectorParamsAs1DForOutWhenUnconnected=off  OutputFunctionCall=on

== system GCI_Ctrl_PLL_C2000/C2000_SW/MnrErr ==
  ADC : Inport
  Irms : Inport  Port=2
  Vdc : Inport  Port=3
  Trigger : TriggerPort  TriggerType=function-call  VariantControl=Variant  PortDimensions=1  OutDataTypeStr=single
  Data Store Read3 : DataStoreRead  DataStoreName=EnaMon  IndexOptions=Index vector (dialog)  Indices=1  OutputSizes=1
  HwFaults : Subsystem
  Monitoring : Subsystem  Priority=2
  OR : Logic  Operator=OR  IconShape=distinctive  AllPortsSameDT=off  OutDataTypeStr=boolean
  Failure : Outport
  FailCodeSw : Outport  Port=2
  FailCodeHw : Outport  Port=3
  wires:
  ADC/1 -> Monitoring/1(ADC)  "ADC"
  Data Store Read3/1 -> Monitoring/Enable
  Monitoring/1(Failure) -> OR/1
  Irms/1 -> Monitoring/2(Irms)  "Irms"
  Vdc/1 -> Monitoring/3(Vdc)  "Vdc"
  Monitoring/2(FailCode) -> FailCodeSw/1
  HwFaults/1(FLT) -> OR/2
  HwFaults/2(FltCodeHw) -> FailCodeHw/1
  OR/1 -> Failure/1

== system GCI_Ctrl_PLL_C2000/C2000_SW/Subsystem ==

== system GCI_Ctrl_PLL_C2000/C2000_SW/SysSts ==
  FrcPwr : Inport
  MdReq : Inport  Port=2
  SysStsFail : Inport  Port=3
  SysStsSynch : Inport  Port=4
  HvdcUAct : Inport  Port=5
  HvacUMinAct : Inport  Port=6
  Trigger : TriggerPort  TriggerType=function-call  VariantControl=Variant  PortDimensions=1  OutDataTypeStr=single
  Data Store Read3 : DataStoreRead  DataStoreName=EnaMon  IndexOptions=Index vector (dialog)  Indices=1  OutputSizes=1
  States : Stateflow chart  TreatAsAtomicUnit=on
  ModAct : Outport
  SafeState : Outport  Port=2
  ControllerEn : Outport  Port=3
  PllEn : Outport  Port=4
  wires:
  FrcPwr/1 -> States/1(FrcPwr)
  MdReq/1 -> States/2(MdReq)
  HvdcUAct/1 -> States/3(HvdcUAct)
  States/1(" StatesMode") -> ModAct/1
  States/2(SafeState) -> SafeState/1
  HvacUMinAct/1 -> States/4(HvacUMinAct)
  SysStsFail/1 -> States/5(SysStsFail)
  SysStsSynch/1 -> States/6(SysStsSynch)
  States/4(PllEn) -> PllEn/1
  States/3(ControllerEn) -> ControllerEn/1
  Data Store Read3/1 -> States/7(EnaMon)

== system GCI_Ctrl_PLL_C2000/PowerSystem/Actual System ==
  DutyIn : Inport
  AC Voltage Source : spsACVoltageSourceLib/AC Voltage Source  Amplitude=double(Var.Grid.VphRms)*sqrt(2)  Phase=0  Frequency=double(Var.Grid.Frq)  SampleTime=0  Measurements=None  BusType=swing  Pref=10e3  Qref=0  Qmin=-inf  Qmax=+inf
  Current Measurement{,1..3} (4 alike) : spsCurrentMeasurementLib/Current Measurement  PhasorSimulation=off  OutputType=Complex  PSBequivalent=0
  Data Type Conversion : DataTypeConversion  SaturateOnIntegerOverflow=off  RndMeth=Floor
  Data Type Conversion1 : DataTypeConversion  SaturateOnIntegerOverflow=off  RndMeth=Floor
  Ground : Ground
  Ground1 : spsGroundLib/Ground  LConnTagsString=a
  Ground2 : spsGroundLib/Ground  LConnTagsString=a
  Measurment : Subsystem
  PWMGen2 : Subsystem  VariantControl=Var.Sim.SimOrHw == 1
  Scope : Scope  NumInputPorts=2
  Series RLC Branch : spsSeriesRLCBranchLib/Series RLC Branch  LConnTagsString=__new0  RConnTagsString=__new0  BranchType=RC  Resistance=double(Var.HVDC.Cesr)  Inductance=1e-3  SetiL0=off  InitialCurrent=0  Capacitance=double(Var.HVDC.C)  Setx0=on  InitialVoltage=double(Var.Grid.VphRms)*sqrt(2)+2  Measurements=Branch voltage and current
  Series RLC Branch1 : spsSeriesRLCBranchLib/Series RLC Branch  LConnTagsString=__new0  RConnTagsString=__new0  BranchType=RL  Resistance=double(Var.HVDC.Lesr)  Inductance=double(Var.HVDC.L)  SetiL0=off  InitialCurrent=0  Capacitance=Var.HVDC.C  Setx0=off  InitialVoltage=0  Measurements=Branch voltage and current
  Terminator : Terminator
  Three-Phase Programmable Voltage Source1 : spsThreePhaseProgrammableVoltageSourceLib/Three-Phase Programmable Voltage Source  PositiveSequence="[double(Var.Grid.VphRms)*sqrt(3)  0 double(Var.Grid.Frq)]"  VariationEntity=None  VariationType=Table of time-amplitude pairs  VariationTypeAlt=Step  VariationStep=-20  VariationRate=10  VariationMagnitude=0.3  VariationFrequency=2  VariationTiming=[1 2]  VariationPhaseA=on  Amplitudes=[1 0.2 1]  TimeValues=[0 0.1 100]  HarmonicGeneration=off  HarmonicA=[3 0.05 -25 0]  HarmonicB=[5 0.05 35 0]  Timing="[0  110]"  BusType=swing  Pref=0  Qref=0  Qmin=-inf  Qmax=inf
  Three-Phase Series RLC Branch : spsThreePhaseSeriesRLCBranchLib/Three-Phase Series RLC Branch  LConnTagsString=A|B|C  RConnTagsString=A|B|C  BranchType=RL  Resistance=double(Var.Inductor.R)  Inductance=double(Var.Inductor.L)  Capacitance=1e-6  Measurements=None
  Three-Phase Transformer (Two Windings) : spsThreePhaseTransformerTwoWindingsLib/Three-Phase Transformer (Two Windings)  Winding1Connection=Yn  Winding2Connection=Yn  CoreType=Three single-phase transformers  SetSaturation=off  Hysteresis=off  DataFile='hysteresis'  SetInitialFlux=off  Measurements=None  UNITS=SI  NominalPower=[ 100e3 , 50 ]  Winding1=[100 Var.Transformer.R1 Var.Transformer.L1]  Winding2=[double(Var.Transformer.N )*100 Var.Transformer.R2*(Var.Transformer.N )^2 Var.Transformer.R2*(Var.Transformer.N )^2]  Rm=Var.Transformer.Rc  Lm=Var.Transformer.Lm  L0=0.5  Saturation=[0 0;1.1327 0.53955;471.96 0.68343]  InitialFluxes=[0.3597 -0.3597 0.31474]  BreakLoop=off  DiscreteSolver=Trapezoidal iterative  DataType=on  TransfoNumber=1
  Three-Phase V-I Measurement1 : spsThreePhaseVIMeasurementLib/Three-Phase V-I Measurement  VoltageMeasurement=phase-to-ground  SetLabelV=on  LabelV=Vgrid_Ls  Vpu=off  VpuLL=off  CurrentMeasurement=no  SetLabelI=off  LabelI=Igrid_Ls  Ipu=off  Pbase=100e6  Vbase=500e3  OutputType=Complex  PhasorSimulation=off  PSBequivalent=0
  Three-Phase V-I Measurement2 : spsThreePhaseVIMeasurementLib/Three-Phase V-I Measurement  VoltageMeasurement=phase-to-ground  SetLabelV=on  LabelV=Vgrid_Hs  Vpu=off  VpuLL=off  CurrentMeasurement=yes  SetLabelI=on  LabelI=Igrid_Hs  Ipu=off  Pbase=100e6  Vbase=500e3  OutputType=Complex  PhasorSimulation=off  PSBequivalent=0
  Three-Phase V-I Measurement4 : spsThreePhaseVIMeasurementLib/Three-Phase V-I Measurement  VoltageMeasurement=phase-to-ground  SetLabelV=on  LabelV=Vinv  Vpu=off  VpuLL=off  CurrentMeasurement=yes  SetLabelI=on  LabelI=Iinv  Ipu=off  Pbase=100e6  Vbase=500e3  OutputType=Complex  PhasorSimulation=off  PSBequivalent=0
  Triggered Subsystem : Subsystem  TreatAsAtomicUnit=on
  Two-Level Converter : spsTwoLevelConverterLib/Two-Level Converter  ModelType=Switching devices  Ron=1e-3  Rs=1e6  Cs=inf  Vforward=[0,0]  Ron_Diode=1e-3  Rs_Diode=1e6  Cs_Diode=inf  Vf_Diode=1e-3  Rs_CurrentSource=inf  Ron_ACsource=1e-3
      settings: LibrarySourceBlock=sps_lib/Power Electronics/Two-Level Converter
  Universal Bridge : spsUniversalBridgeLib/Universal Bridge  Arms=2  SnubberResistance=1e5  SnubberCapacitance=inf  Device=Diodes  Ron=1e-3  Lon=0  ForwardVoltages="[  0  0  ]"  ForwardVoltage=0  GTOparameters=[ 10e-6 , 20e-6 ]  IGBTparameters=[ 1e-6 , 2e-6 ]  Measurements=None  Measurements_2=None  converterType=Rectifier
  Voltage Measurement : spsVoltageMeasurementLib/Voltage Measurement  PhasorSimulation=off  OutputType=Complex  PSBequivalent=0
  Voltage Measurement1 : spsVoltageMeasurementLib/Voltage Measurement  PhasorSimulation=off  OutputType=Complex  PSBequivalent=0
  Voltage Measurement2 : spsVoltageMeasurementLib/Voltage Measurement  PhasorSimulation=off  OutputType=Complex  PSBequivalent=0
  powergui1 : spspowerguiLib/powergui  Priority=1  SimulationMode=Discrete  SampleTime=Sim.ContSampleTime  frequency=60  Iterations=50  frequencyindice=0  Pbase=100e6  ErrMax=1e-4  UnitsV=kV  UnitsW=MW  buscounter=0  FunctionMessages=off  echomessages=off  EnableUseOfTLC=off  CurrentSourceSwitches=off  DisableSnubberDevices=off  DisableRonSwitches=off  DisableVfSwitches=off  DisplayEquations=off  AutomaticDiscreteSolvers=off  SolverType=Tustin/Backward Euler (TBE)  Interpol=off  ExternalGateDelay=off  methode=off  Ts=100  x0status=blocks  SPID=off  SwTol=0  HookPort=off  NonlinearTolerance=1e-4  nMaxIteration=100  ContinueOnMaxIteration=off  RestoreLinks=warning  ResistiveCurrentMeasurement=off  Frange=[0:2:500]  Ylog=off  Xlog=on  ShowGrid=off  save=off  variable=ZData  structure=ScopeData2  ZoomFFT=off  StartTime=4.2  cycles=50  DisplayStyle=3  fundamental=46.5  FreqAxis=on  MaxFrequency=inf  frequencyindicesteady=1  RmsSteady=1  display=off
  MCU : Outport  VectorParamsAs1DForOutWhenUnconnected=off
  wires:
  PWMGen2/1(PWM) -> Data Type Conversion1/1
  Current Measurement2/1 -> [Ibridge]
  [Iinv] -> Measurment/5(Iinv_abc)
  Voltage Measurement1/1 -> [Vhvdc]
  Current Measurement/1 -> [Ihvdc]
  Ground/1 -> Two-Level Converter/2
  Data Type Conversion1/1 -> [PWM], Two-Level Converter/1
  DutyIn/1 -> PWMGen2/1(Duty)
  [Vgrid_Ls] -> Measurment/3(Vgrid_abc)
  [Vhvdc] -> Measurment/6(V_HVDC)
  [Ihvdc] -> Measurment/7(I_HVDC)
  Measurment/1(MCU) -> Data Type Conversion/1
  [Vinv] -> Measurment/4(Vinv_abc)
  [Ibridge] -> Measurment/10(Ibridge)
  Current Measurement1/1 -> [IhvdcCap]
  Data Type Conversion/1 -> Scope/1, Triggered Subsystem/1(In1)
  Voltage Measurement/1 -> [Vbridge]
  [IhvdcCap] -> Measurment/8(Ihvdc_capa)
  [Vbridge] -> Measurment/9(Vbdg)
  [Igrid_Hs] -> Measurment/2(Igrid_abc_HS)
  [Vgrid_Hs] -> Measurment/1(Vgrid_abc_HS)
  Voltage Measurement2/1 -> [Vbridge_In]
  Current Measurement3/1 -> [Ibridge_In]
  [Vbridge_In] -> Measurment/11(VbridgeIn)
  [Ibridge_In] -> Measurment/12(IbridgeIn)
  [PWM] -> Measurment/13(In13)
  Measurment/2(Meas) -> Terminator/1
  Triggered Subsystem/1(Out1) -> Scope/2, MCU/1
  PWMGen2/2(MeasTrig) -> [Trig]
  [Trig] -> Triggered Subsystem/Trigger
  connections:
  Voltage Measurement2/LConn2 -- Universal Bridge/LConn2 -- AC Voltage Source/LConn1
  Three-Phase Transformer (Two Windings)/LConn2 -- Three-Phase V-I Measurement1/LConn2
  Three-Phase V-I Measurement4/RConn3 -- Three-Phase Series RLC Branch/LConn3
  Current Measurement1/RConn1 -- Series RLC Branch/LConn1
  Three-Phase V-I Measurement4/LConn2 -- Two-Level Converter/LConn2
  Three-Phase V-I Measurement4/LConn1 -- Two-Level Converter/LConn1
  Current Measurement2/RConn1 -- Voltage Measurement1/LConn1 -- Current Measurement/LConn1 -- Current Measurement1/LConn1
  Voltage Measurement/LConn1 -- Universal Bridge/RConn1 -- Series RLC Branch1/LConn1
  Current Measurement2/LConn1 -- Series RLC Branch1/RConn1
  Three-Phase V-I Measurement1/RConn2 -- Three-Phase Series RLC Branch/RConn2
  Three-Phase V-I Measurement1/RConn3 -- Three-Phase Series RLC Branch/RConn3
  Three-Phase V-I Measurement4/RConn2 -- Three-Phase Series RLC Branch/LConn2
  Three-Phase V-I Measurement4/LConn3 -- Two-Level Converter/LConn3
  Current Measurement/RConn1 -- Two-Level Converter/RConn1
  Two-Level Converter/RConn2 -- Series RLC Branch/RConn1 -- Voltage Measurement/LConn2 -- Voltage Measurement1/LConn2 -- Universal Bridge/RConn2
  Three-Phase V-I Measurement1/RConn1 -- Three-Phase Series RLC Branch/RConn1
  Three-Phase V-I Measurement4/RConn1 -- Three-Phase Series RLC Branch/LConn1
  Three-Phase V-I Measurement1/LConn1 -- Three-Phase Transformer (Two Windings)/LConn1
  Three-Phase V-I Measurement1/LConn3 -- Three-Phase Transformer (Two Windings)/LConn3
  Current Measurement3/RConn1 -- Universal Bridge/LConn1
  Current Measurement3/LConn1 -- AC Voltage Source/RConn1 -- Voltage Measurement2/LConn1
  Three-Phase Transformer (Two Windings)/RConn4 -- Ground2/LConn1 -- Three-Phase Programmable Voltage Source1/LConn1
  Ground1/LConn1 -- Three-Phase Transformer (Two Windings)/LConn4
  Three-Phase V-I Measurement2/LConn1 -- Three-Phase Transformer (Two Windings)/RConn1
  Three-Phase V-I Measurement2/LConn2 -- Three-Phase Transformer (Two Windings)/RConn2
  Three-Phase V-I Measurement2/LConn3 -- Three-Phase Transformer (Two Windings)/RConn3
  Three-Phase V-I Measurement2/RConn3 -- Three-Phase Programmable Voltage Source1/RConn3
  Three-Phase V-I Measurement2/RConn2 -- Three-Phase Programmable Voltage Source1/RConn2
  Three-Phase V-I Measurement2/RConn1 -- Three-Phase Programmable Voltage Source1/RConn1

== system GCI_Ctrl_PLL_C2000/PowerSystem/HW ==
  DutyIn : Inport
  Ground{,1..5} (6 alike) : Ground
  Mux : Mux  Inputs=6
  Terminator : Terminator
  MCU : Outport  VectorParamsAs1DForOutWhenUnconnected=off
  wires:
  DutyIn/1 -> Terminator/1
  Mux/1 -> MCU/1
  Ground1/1 -> Mux/2
  Ground/1 -> Mux/1
  Ground2/1 -> Mux/3
  Ground3/1 -> Mux/4
  Ground5/1 -> Mux/6
  Ground4/1 -> Mux/5

== system GCI_Ctrl_PLL_C2000/PowerSystem/Meas ==
  DutyIn : Inport
  Constant3 : Constant  Value=[Var.ADC.CH0.PHY_OFFSET Var.ADC.CH1.PHY_OFFSET Var.ADC.CH4.PHY_OFFSET]
  Demux : Demux  Outputs=3
  Fault Injection : Subsystem  Variant=on  VariantControl=Variant1
  Ia : Sin  Amplitude=2.26  Bias=1.58  Frequency=2*pi*46.5  SampleTime=1/double(Var.PWM.Freq)
  Ib : Sin  Amplitude=2.24  Bias=1.68  Frequency=2*pi*46.5  Phase=(7.12/21.5)*2*pi  SampleTime=1/double(Var.PWM.Freq)
  Mux : Mux  Inputs=6
  Sum : Sum  Inputs=++|
  Terminator : Terminator
  Vdc : Sin  Amplitude=0.1  Bias=1.68  Frequency=2*pi*46.5  Phase=(7.12/21.5)*2*pi  SampleTime=1/double(Var.PWM.Freq)
  MCU : Outport  VectorParamsAs1DForOutWhenUnconnected=off
  wires:
  Ib/1 -> Mux/5
  Ia/1 -> Mux/4
  DutyIn/1 -> Terminator/1
  Vdc/1 -> Mux/6
  Sum/1 -> Demux/1
  Demux/1 -> Mux/1
  Demux/2 -> Mux/2
  Demux/3 -> Mux/3
  Fault Injection/1(Wave) -> Sum/2
  Mux/1 -> MCU/1
  Constant3/1 -> Sum/1
